simulink model "On_off_model"  (Simulink 7.8)
settings: Solver=ode3  StartTime=0.0  StopTime=5500  FixedStep=1  RelTol=1e-3
undefined symbols (not defined in the file or in its folder): sys
settings Model: Creator=Lenovo  LastModifiedBy=Lenovo

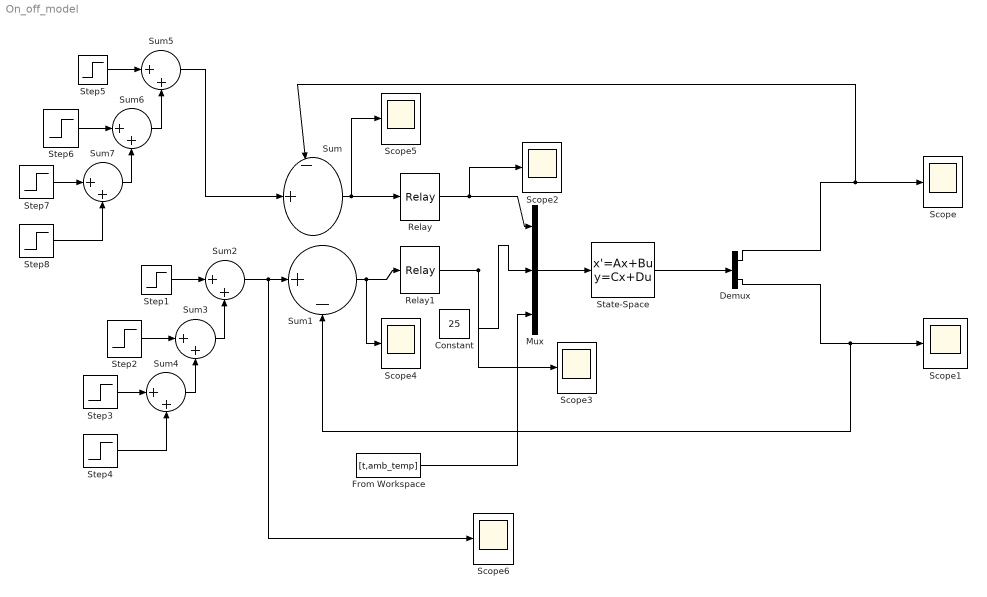
== system On_off_model ==
  Constant : Constant  Value=25
  Demux : Demux  Outputs=2
  From Workspace : FromWorkspace  VariableName=[t,amb_temp]  SampleTime=0
  Mux : Mux  Inputs=3
  Relay : Relay  OnSwitchValue=1  OffSwitchValue=-1  OnOutputValue=40  OffOutputValue=15
  Relay1 : Relay  OnSwitchValue=1  OffSwitchValue=-1  OnOutputValue=40  OffOutputValue=15
  Scope{,1..6} (7 alike) : Scope
      Scope settings: SaveName=NBT  DataFormat=Array  MaxDataPoints=5500
      Scope1 settings: SaveName=SBT  DataFormat=Array  MaxDataPoints=5500
      Scope2 settings: SaveName=swn  DataFormat=Array  MaxDataPoints=5500
      Scope3 settings: SaveName=sws  DataFormat=Array  MaxDataPoints=5500
      Scope4 settings: SaveName=ScopeData4
      Scope5 settings: SaveName=ScopeData5
      Scope6 settings: SaveName=ScopeData6
  State-Space : StateSpace  A=sys.a  B=sys.b  C=sys.c  D=sys.d  X0=[26 28 23 23.5]  ContinuousStateAttributes='Temperature'
  Step1 : Step  Time=1000  Before=20  After=25  SampleTime=0
  Step2 : Step  Time=2000  After=-3  SampleTime=0
  Step3 : Step  Time=3000  After=4  SampleTime=0
  Step4 : Step  Time=4000  After=-3  SampleTime=0
  Step5 : Step  Time=1000  Before=20  After=25  SampleTime=0
  Step6 : Step  Time=2000  After=-3  SampleTime=0
  Step7 : Step  Time=3000  After=4  SampleTime=0
  Step8 : Step  Time=4000  After=-3  SampleTime=0
  Sum : Sum  Inputs=|-||||+||||||
  Sum1 : Sum  Inputs=|+-
  Sum{2..7} (6 alike) : Sum  Inputs=|++
  wires:
  Relay/1 -> Mux/1, Scope2/1
  State-Space/1 -> Demux/1
  Demux/1 -> Scope/1, Sum/1
  Demux/2 -> Scope1/1, Sum1/2
  Relay1/1 -> Scope3/1, Mux/2
  Sum1/1 -> Relay1/1, Scope4/1
  Sum/1 -> Relay/1, Scope5/1
  Mux/1 -> State-Space/1
  Sum2/1 -> Sum1/1, Scope6/1
  Step1/1 -> Sum2/1
  Sum3/1 -> Sum2/2
  Step2/1 -> Sum3/1
  Sum4/1 -> Sum3/2
  Step3/1 -> Sum4/1
  Step4/1 -> Sum4/2
  Step5/1 -> Sum5/1
  Sum6/1 -> Sum5/2
  Step6/1 -> Sum6/1
  Sum7/1 -> Sum6/2
  Step7/1 -> Sum7/1
  Step8/1 -> Sum7/2
  Sum5/1 -> Sum/2
  From Workspace/1 -> Mux/3
